simulink model "gm_sampleModel1467_3_sub"  (R2023a)
settings: Solver=VariableStepAuto  StartTime=0.0  StopTime=10.0  RelTol=1e-3
libraries: simulink x1
settings Model: Creator=user1  LastModifiedBy=user1
settings OptimizationCC: BlockReduction=off  ConditionallyExecuteInputs=off
settings DebuggingCC: InheritedTsInSrcMsg=none

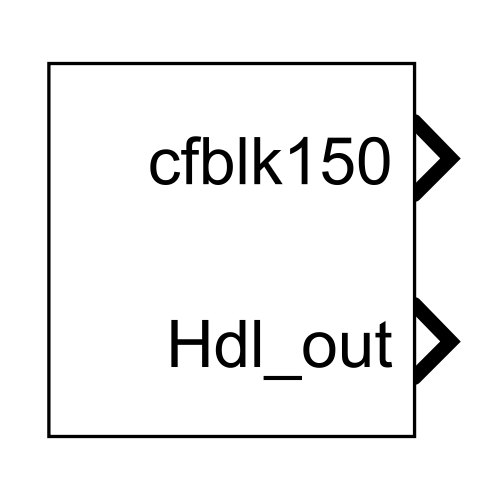
[thumbnail: Simulink's stored preview of the top-level diagram]
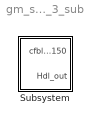
== system gm_sampleModel1467_3_sub ==
  Subsystem : Subsystem

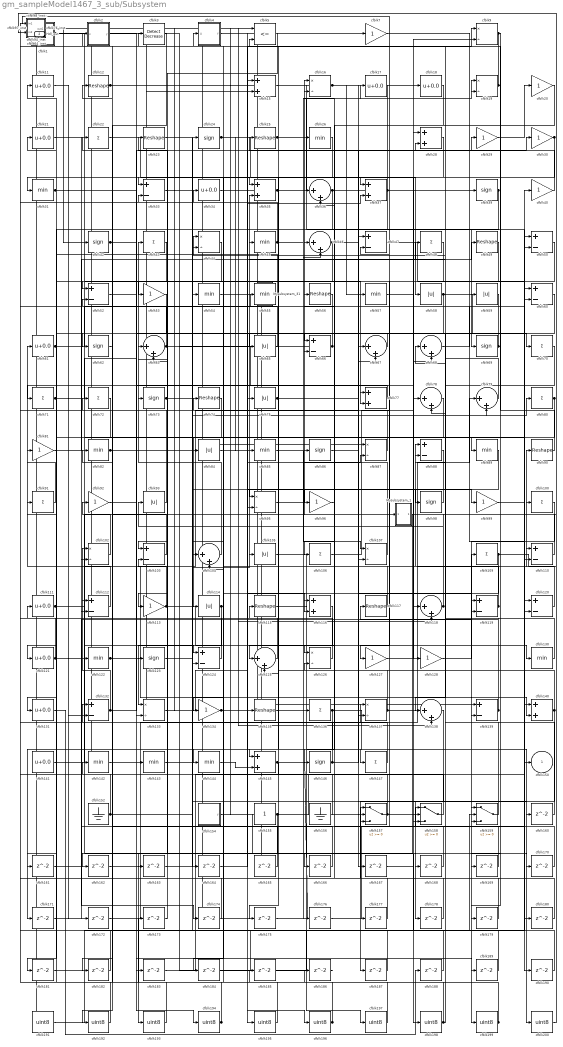
== system gm_sampleModel1467_3_sub/Subsystem ==
  Mysubsystem_1 : Subsystem
  Mysubsystem_31 : Subsystem
  cfblk1 : Subsystem  mask(Compare To Constant){relop=<=, const=double(3), OutDataTypeStr=uint8, ZeroCross=on}
      mask prompts: relop "Simulink:masks:Operator_MP"; const "Simulink:masks:ConstantValue_MP"; OutDataTypeStr "Simulink:masks:OutputDataType_MP"; ZeroCross "Simulink:masks:EnableZerocrossingDetection_MP"
      mask help: Simulink:masks:CompareToConstant_MD
      mask init:
      | OutDataTypeStr = 'uint8';
      | ZeroCross = 'on';
      | blkName = 'sampleModel1467_3_sub/Subsystem/cfblk1';
      | const = double(3);
      | const_str = '3.0';
      | const_val = double(3);
      | relop = '<=';
      | setValue = 'fixdt(0, 8)';
      | str = '<= 3';
      mask TypeOptions relop: == | ~= | < | <= | >= | >
      mask TypeOptions OutDataTypeStr: Simulink:masks:uint8 | Simulink:masks:boolean
      mask Callback ZeroCross: sl('zeroCrossEnable', gcbh);
      mask Display: disp(str)
  cfblk{22,43,48,70..72,80,91,100,106,109,136,147} (13 alike) : Sum  Inputs=+  OutDataTypeStr=uint8
  cfblk101_inst : Subsystem
  cfblk{9,16,19,44,87,95,102,107,126,133,137} (11 alike) : Product  Inputs=*/  OutDataTypeStr=uint8  RndMeth=Zero  SaturateOnIntegerOverflow=on
  cfblk{33,47,50,52,60,66,88,103,110,112,119..120,124,132,139} (15 alike) : Sum  Inputs=+-  OutDataTypeStr=uint8
  cfblk{36,46,63,67..68,78..79,104,118,125,138} (11 alike) : Sum  Inputs=|++  OutDataTypeStr=uint8
  cfblk{58..59,65,75,84,93,105,114} (8 alike) : Abs  OutDataTypeStr=uint8  SaturateOnIntegerOverflow=off
  cfblk{11,17..18,21,34,61,111,121,131,141} (10 alike) : Bias  Bias=0.0  SaturateOnIntegerOverflow=off
  cfblk{7,20,29..30,40,53,81,92,96,99,113,127..128,134} (14 alike) : Gain  OutDataTypeStr=uint8
  cfblk{12,23,25,49,56,74,90,115,117,135} (10 alike) : Reshape
  cfblk{15,28,35,37,77,116,140,145} (8 alike) : Sum  OutDataTypeStr=uint8
  cfblk{26,31,45,54..55,57,82,85,89,122,130,142..144} (14 alike) : MinMax  OutDataTypeStr=uint8
  cfblk{24,39,42,62,69,73,86,98,123,146} (10 alike) : Signum
  cfblk13_inst : Subsystem
  cfblk14_inst : Subsystem
  cfblk152 : Ground
  cfblk154 : Subsystem  mask(Counter Free-Running){NumBits=double(16), tsamp=double(-1)}
      mask prompts: NumBits "Simulink:masks:NumberOfBits_MP"; tsamp "Simulink:masks:SampleTime_MP"
      mask help: Simulink:masks:CounterFreeRunning_MD
  cfblk155 : Constant  OutDataTypeStr=uint8  SampleTime=-1
  cfblk156 : Ground
  cfblk157 : Switch  OutDataTypeStr=uint8  SaturateOnIntegerOverflow=off  InputSameDT=off
  cfblk158 : Switch  OutDataTypeStr=uint8  SaturateOnIntegerOverflow=off  InputSameDT=off
  cfblk159 : Switch  OutDataTypeStr=uint8  SaturateOnIntegerOverflow=off  InputSameDT=off
  cfblk{160..190} (31 alike) : Delay  SampleTime=1
  cfblk{191..200} (10 alike) : DataTypeConversion  OutDataTypeStr=uint8  SaturateOnIntegerOverflow=off  RndMeth=Floor
  cfblk2 : Subsystem  mask(Compare To Constant){relop=<=, const=double(3), OutDataTypeStr=uint8, ZeroCross=on}
      mask prompts: relop "Simulink:masks:Operator_MP"; const "Simulink:masks:ConstantValue_MP"; OutDataTypeStr "Simulink:masks:OutputDataType_MP"; ZeroCross "Simulink:masks:EnableZerocrossingDetection_MP"
      mask help: Simulink:masks:CompareToConstant_MD
      mask init:
      | OutDataTypeStr = 'uint8';
      | ZeroCross = 'on';
      | blkName = 'sampleModel1467_3_sub/Subsystem/cfblk2';
      | const = double(3);
      | const_str = '3.0';
      | const_val = double(3);
      | relop = '<=';
      | setValue = 'fixdt(0, 8)';
      | str = '<= 3';
      mask TypeOptions relop: == | ~= | < | <= | >= | >
      mask TypeOptions OutDataTypeStr: Simulink:masks:uint8 | Simulink:masks:boolean
      mask Callback ZeroCross: sl('zeroCrossEnable', gcbh);
      mask Display: disp(str)
  cfblk3 : simulink/Logic and Bit Operations/Detect Decrease  vinit=0.0  OutDataTypeStr=uint8
      settings: LibrarySourceBlock=|
      | hdlsllib/Logic and Bit
      | Operations/Detect
      | Decrease
  cfblk32_inst : Subsystem
  cfblk38_inst : Subsystem
  cfblk4 : Subsystem  mask(Detect Fall Nonpositive){vinit=double(0), InputProcessing=Elements as channels (sample based), OutDataTypeStr=uint8}
      mask prompts: vinit "Simulink:masks:InitialCondition_MP"; InputProcessing "Simulink:masks:InputProcessing_MP"; OutDataTypeStr "Simulink:masks:OutputDataType_MP"
      mask help: Simulink:masks:DetectFallNonpositive_MD
      mask init:
      | InputProcessing = 'Elements as channels (sample based)';
      | OutDataTypeStr = 'uint8';
      | vinit = double(0);
      mask TypeOptions InputProcessing: Simulink:masks:ColumnsAsChannelsFrameBased | Simulink:masks:ElementsAsChannelsSampleBased
      mask TypeOptions OutDataTypeStr: Simulink:masks:uint8 | Simulink:masks:boolean
      mask Display: fprintf('U <= 0\n&  NOT\nU/z <= 0')
  cfblk41_inst : Subsystem
  cfblk5 : RelationalOperator  Operator=<=  OutDataTypeStr=boolean  InputSameDT=off
  cfblk51_inst : Subsystem
  cfblk64_inst : Subsystem
  cfblk6_inst : Subsystem
  cfblk76_inst : Subsystem
  cfblk8_inst : Subsystem
  cfblk94_inst : Subsystem
  cfblk97_inst : Subsystem
  cfblk150 : Outport  OutDataTypeStr=uint8  SampleTime=1  VectorParamsAs1DForOutWhenUnconnected=off
  Hdl_out : Outport  Port=2  OutDataTypeStr=uint8  SampleTime=1
  wires:
  Mysubsystem_1/1(Out1) -> cfblk162/1
  Mysubsystem_31/1(Out1) -> cfblk165/1
  cfblk1/1(y) -> cfblk77/2, cfblk124/1
  cfblk100/1 -> cfblk199/1
  cfblk101_inst/1(out1) -> cfblk15/2, cfblk135/1
  cfblk102/1 -> cfblk92/1
  cfblk103/1 -> cfblk12/1
  cfblk104/1 -> cfblk43/1
  cfblk105/1 -> cfblk197/1
  cfblk106/1 -> cfblk14_inst/1(in1)
  cfblk107/1 -> cfblk16/1
  cfblk109/1 -> cfblk14_inst/2(in2), cfblk144/1
  cfblk11/1 -> cfblk172/1
  cfblk110/1 -> cfblk74/1
  cfblk111/1 -> cfblk66/2, cfblk200/1
  cfblk112/1 -> cfblk61/1
  cfblk113/1 -> cfblk103/2, cfblk130/1
  cfblk114/1 -> cfblk34/1, cfblk133/1
  cfblk115/1 -> cfblk147/1
  cfblk116/1 -> cfblk125/1
  cfblk117/1 -> cfblk35/2
  cfblk118/1 -> cfblk93/1, cfblk6_inst/2(in2)
  cfblk119/1 -> cfblk88/1, cfblk56/1, cfblk13_inst/1(in1)
  cfblk12/1 -> cfblk116/2, cfblk89/1
  cfblk120/1 -> cfblk90/1
  cfblk121/1 -> cfblk8_inst/1(in1), cfblk67/2
  cfblk122/1 -> cfblk47/1, cfblk139/2
  cfblk123/1 -> cfblk105/1
  cfblk124/1 -> cfblk38_inst/1(in1)
  cfblk125/1 -> cfblk22/1
  cfblk126/1 -> cfblk82/1
  cfblk127/1 -> cfblk68/2
  cfblk128/1 -> cfblk109/1
  cfblk13_inst/1(out1) -> cfblk7/1, cfblk136/1
  cfblk130/1 -> cfblk3/1
  cfblk131/1 -> cfblk188/1
  cfblk132/1 -> cfblk102/1, Mysubsystem_31/1(In1)
  cfblk133/1 -> cfblk55/1
  cfblk134/1 -> cfblk37/2, cfblk30/1
  cfblk135/1 -> cfblk17/1
  cfblk136/1 -> cfblk171/1, cfblk170/1
  cfblk137/1 -> cfblk79/1, cfblk46/1
  cfblk138/1 -> cfblk187/1
  cfblk139/1 -> cfblk117/1, cfblk44/1
  cfblk14_inst/1(out1) -> cfblk138/2
  cfblk140/1 -> cfblk73/1, cfblk178/1
  cfblk141/1 -> cfblk24/1
  cfblk142/1 -> cfblk86/1
  cfblk143/1 -> cfblk160/1
  cfblk144/1 -> cfblk145/2
  cfblk145/1 -> cfblk176/1, cfblk175/1
  cfblk146/1 -> cfblk5/2, cfblk29/1
  cfblk147/1 -> cfblk64_inst/2(in2)
  cfblk15/1 -> cfblk180/1
  cfblk152/1 -> cfblk8_inst/2(in2), cfblk124/2
  cfblk154/1(y) -> cfblk198/1
  cfblk155/1 -> cfblk193/1, cfblk40/1
  cfblk156/1 -> cfblk51_inst/1(in1)
  cfblk157/1 -> cfblk15/1, cfblk115/1
  cfblk158/1 -> cfblk142/1
  cfblk159/1 -> cfblk94_inst/1(in1)
  cfblk16/1 -> cfblk159/3, cfblk57/1
  cfblk160/1 -> cfblk126/2
  cfblk161/1 -> cfblk158/1
  cfblk162/1 -> cfblk107/2
  cfblk163/1 -> cfblk60/2
  cfblk164/1 -> cfblk87/2
  cfblk165/1 -> cfblk132/1
  cfblk166/1 -> cfblk63/1
  cfblk167/1 -> cfblk78/1
  cfblk168/1 -> cfblk36/2
  cfblk169/1 -> cfblk157/1
  cfblk17/1 -> cfblk33/1
  cfblk170/1 -> cfblk47/2
  cfblk171/1 -> cfblk119/2
  cfblk172/1 -> cfblk110/1
  cfblk173/1 -> cfblk33/2
  cfblk174/1 -> cfblk52/2
  cfblk175/1 -> cfblk137/1
  cfblk176/1 -> cfblk120/2
  cfblk177/1 -> cfblk94_inst/2(in2)
  cfblk178/1 -> cfblk157/3
  cfblk179/1 -> cfblk16/2
  cfblk18/1 -> cfblk146/1
  cfblk180/1 -> cfblk64_inst/1(in1)
  cfblk181/1 -> cfblk50/1
  cfblk182/1 -> cfblk41_inst/2(in2)
  cfblk183/1 -> cfblk46/2
  cfblk184/1 -> cfblk159/2
  cfblk185/1 -> cfblk158/3
  cfblk186/1 -> cfblk1/1(u)
  cfblk187/1 -> cfblk112/1
  cfblk188/1 -> cfblk32_inst/1(in1)
  cfblk189/1 -> cfblk38_inst/2(in2)
  cfblk19/1 -> cfblk13_inst/2(in2), cfblk169/1
  cfblk190/1 -> cfblk68/1
  cfblk191/1 -> cfblk54/1
  cfblk192/1 -> cfblk97_inst/1(in1)
  cfblk193/1 -> cfblk97_inst/2(in2)
  cfblk194/1 -> cfblk11/1, cfblk173/1
  cfblk195/1 -> cfblk2/1(u)
  cfblk196/1 -> cfblk111/1, cfblk186/1
  cfblk197/1 -> cfblk4/1(U)
  cfblk198/1 -> cfblk88/2, cfblk76_inst/2(in2)
  cfblk199/1 -> cfblk185/1, cfblk91/1
  cfblk2/1(y) -> cfblk194/1
  cfblk20/1 -> cfblk137/2
  cfblk200/1 -> cfblk100/1
  cfblk21/1 -> cfblk174/1
  cfblk22/1 -> cfblk75/1
  cfblk23/1 -> cfblk140/2
  cfblk24/1 -> cfblk58/1, cfblk128/1, cfblk85/1
  cfblk25/1 -> cfblk67/1, cfblk28/2
  cfblk26/1 -> cfblk145/1
  cfblk28/1 -> cfblk37/1
  cfblk29/1 -> cfblk20/1
  cfblk3/1 -> cfblk192/1
  cfblk30/1 -> cfblk104/2, cfblk163/1
  cfblk31/1 -> cfblk183/1, cfblk122/1
  cfblk32_inst/1(out1) -> cfblk18/1, cfblk118/2
  cfblk33/1 -> cfblk35/1
  cfblk34/1 -> cfblk195/1
  cfblk35/1 -> cfblk69/1, cfblk19/1
  cfblk36/1 -> cfblk63/2, cfblk44/2, cfblk133/2, Mysubsystem_1/1(In1)
  cfblk37/1 -> cfblk184/1, cfblk31/1
  cfblk38_inst/1(out1) -> cfblk141/1
  cfblk39/1 -> cfblk121/1, cfblk116/1
  cfblk4/1(Y) -> cfblk196/1
  cfblk40/1 -> cfblk25/1
  cfblk41_inst/1(out1) -> cfblk5/1, cfblk36/1
  cfblk42/1 -> cfblk189/1, cfblk70/1
  cfblk43/1 -> cfblk52/1
  cfblk44/1 -> cfblk181/1
  cfblk45/1 -> cfblk51_inst/2(in2), cfblk19/2
  cfblk46/1 -> cfblk119/1, cfblk102/2
  cfblk47/1 -> cfblk120/1
  cfblk48/1 -> cfblk134/1
  cfblk49/1 -> cfblk96/1
  cfblk5/1 -> cfblk53/1
  cfblk50/1 -> cfblk127/1
  cfblk51_inst/1(out1) -> cfblk177/1
  cfblk52/1 -> cfblk77/1
  cfblk53/1 -> cfblk161/1
  cfblk54/1 -> cfblk9/1
  cfblk55/1 -> cfblk21/1
  cfblk56/1 -> cfblk123/1
  cfblk57/1 -> cfblk9/2
  cfblk58/1 -> cfblk140/1, cfblk125/2, cfblk113/1
  cfblk59/1 -> cfblk78/2
  cfblk6_inst/1(out1) -> cfblk39/1
  cfblk60/1 -> cfblk126/1
  cfblk61/1 -> cfblk50/2, cfblk150/1
  cfblk62/1 -> cfblk182/1
  cfblk63/1 -> cfblk32_inst/2(in2), cfblk118/1
  cfblk64_inst/1(out1) -> cfblk42/1, cfblk87/1
  cfblk65/1 -> cfblk23/1
  cfblk66/1 -> cfblk65/1, Hdl_out/1
  cfblk67/1 -> cfblk62/1
  cfblk68/1 -> cfblk60/1
  cfblk69/1 -> cfblk66/1, cfblk179/1
  cfblk7/1 -> cfblk110/2
  cfblk70/1 -> cfblk138/1
  cfblk71/1 -> cfblk28/1, cfblk132/2, cfblk164/1
  cfblk72/1 -> cfblk131/1
  cfblk73/1 -> cfblk98/1, cfblk79/2, cfblk103/1
  cfblk74/1 -> cfblk114/1
  cfblk75/1 -> cfblk168/1, cfblk167/1
  cfblk76_inst/1(out1) -> cfblk6_inst/1(in1)
  cfblk77/1 -> cfblk71/1
  cfblk78/1 -> cfblk84/1
  cfblk79/1 -> cfblk45/1
  cfblk8_inst/1(out1) -> cfblk139/1, cfblk101_inst/1(in1)
  cfblk80/1 -> cfblk112/2, cfblk104/1
  cfblk81/1 -> cfblk48/1
  cfblk82/1 -> cfblk159/1, cfblk99/1
  cfblk84/1 -> cfblk80/1
  cfblk85/1 -> cfblk107/1
  cfblk86/1 -> cfblk157/2
  cfblk87/1 -> cfblk41_inst/1(in1)
  cfblk88/1 -> cfblk106/1
  cfblk89/1 -> cfblk95/1
  cfblk9/1 -> cfblk59/1, cfblk101_inst/2(in2)
  cfblk90/1 -> cfblk76_inst/1(in1)
  cfblk91/1 -> cfblk81/1
  cfblk92/1 -> cfblk166/1
  cfblk93/1 -> cfblk72/1
  cfblk94_inst/1(out1) -> cfblk158/2, cfblk143/1
  cfblk95/1 -> cfblk49/1
  cfblk96/1 -> cfblk26/1
  cfblk97_inst/1(out1) -> cfblk191/1
  cfblk98/1 -> cfblk95/2
  cfblk99/1 -> cfblk190/1

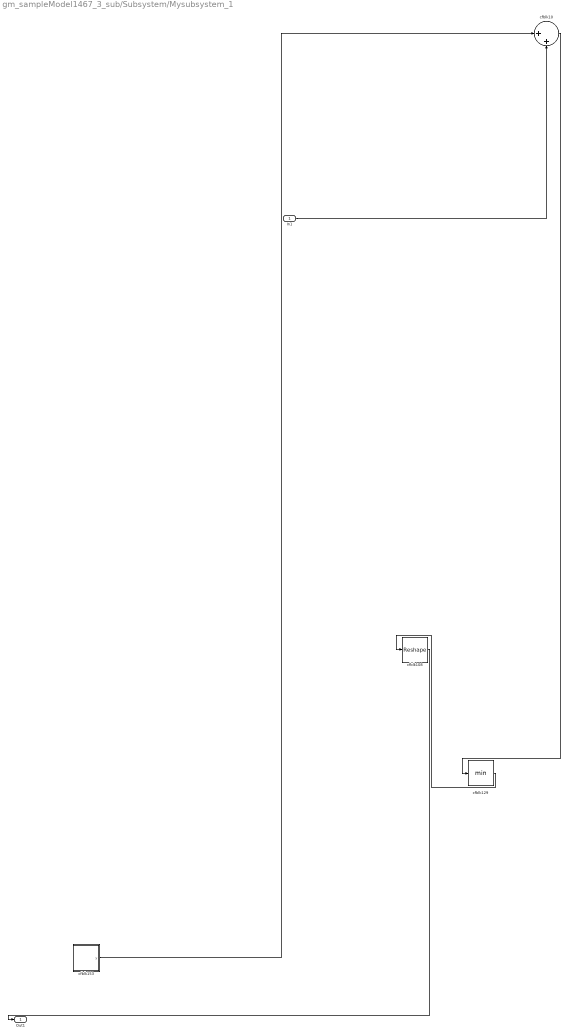
== system gm_sampleModel1467_3_sub/Subsystem/Mysubsystem_1 ==
  In1 : Inport  OutDataTypeStr=uint8  PortDimensions=1  SampleTime=1
  cfblk10 : Sum  Inputs=|++
  cfblk108 : Reshape
  cfblk129 : MinMax
  cfblk153 : Subsystem  mask(Counter Free-Running){NumBits=double(16), tsamp=double(-1)}
      mask prompts: NumBits "Simulink:masks:NumberOfBits_MP"; tsamp "Simulink:masks:SampleTime_MP"
      mask help: Simulink:masks:CounterFreeRunning_MD
  Out1 : Outport  SampleTime=1
  wires:
  In1/1 -> cfblk10/2
  cfblk10/1 -> cfblk129/1
  cfblk108/1 -> Out1/1
  cfblk129/1 -> cfblk108/1
  cfblk153/1(y) -> cfblk10/1

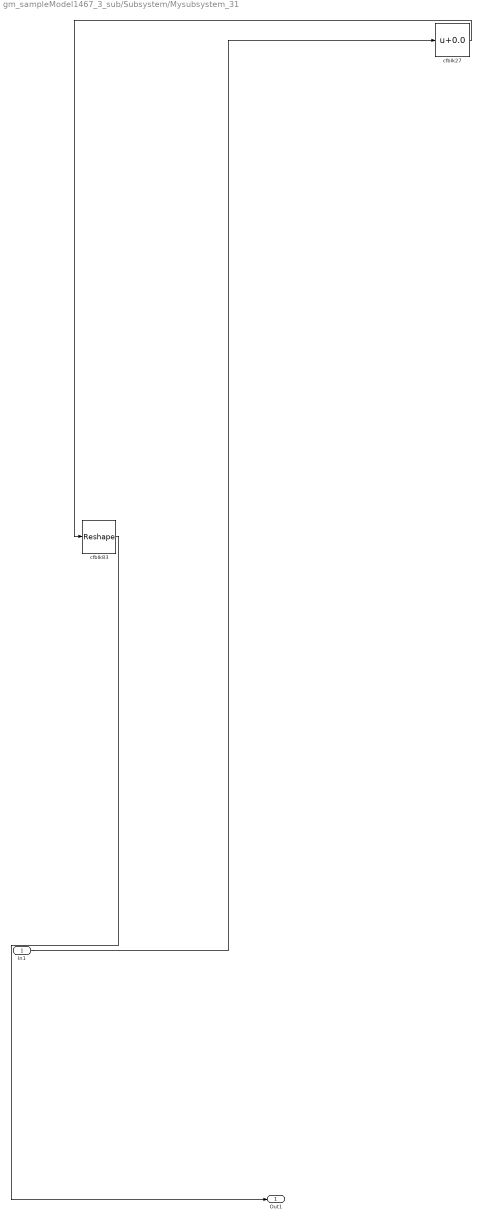
== system gm_sampleModel1467_3_sub/Subsystem/Mysubsystem_31 ==
  In1 : Inport  OutDataTypeStr=uint8  PortDimensions=1  SampleTime=1
  cfblk27 : Bias  Bias=0.0  SaturateOnIntegerOverflow=off
  cfblk83 : Reshape
  Out1 : Outport  SampleTime=1
  wires:
  In1/1 -> cfblk27/1
  cfblk27/1 -> cfblk83/1
  cfblk83/1 -> Out1/1

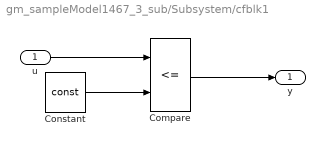
== system gm_sampleModel1467_3_sub/Subsystem/cfblk1 ==
  u : Inport  OutDataTypeStr=uint8  SampleTime=1
  Compare : RelationalOperator  Operator=<=  OutDataTypeStr=fixdt(0, 8)
  Constant : Constant  DisableCoverage=on  Value=const  OutDataTypeStr=Inherit: Inherit via back propagation  SampleTime=-1
  y : Outport  SampleTime=1
  wires:
  u/1 -> Compare/1
  Compare/1 -> y/1
  Constant/1 -> Compare/2

== system gm_sampleModel1467_3_sub/Subsystem/cfblk101_inst ==
  in1 : Inport  OutDataTypeStr=uint8  SampleTime=1
  in2 : Inport  Port=2  OutDataTypeStr=uint8  SampleTime=1
  mul_cfblk101_dotp_mulcomp : Product  Inputs=**  OutDataTypeStr=uint8  SampleTime=1
  out1 : Outport  OutDataTypeStr=uint8  SampleTime=1
  wires:
  in1/1 -> mul_cfblk101_dotp_mulcomp/1
  in2/1 -> mul_cfblk101_dotp_mulcomp/2
  mul_cfblk101_dotp_mulcomp/1 -> out1/1

== system gm_sampleModel1467_3_sub/Subsystem/cfblk13_inst ==
  in1 : Inport  OutDataTypeStr=uint8  SampleTime=1
  in2 : Inport  Port=2  OutDataTypeStr=uint8  SampleTime=1
  mul_cfblk13_dotp_mulcomp : Product  Inputs=**  OutDataTypeStr=uint8  SampleTime=1
  out1 : Outport  OutDataTypeStr=uint8  SampleTime=1
  wires:
  in1/1 -> mul_cfblk13_dotp_mulcomp/1
  in2/1 -> mul_cfblk13_dotp_mulcomp/2
  mul_cfblk13_dotp_mulcomp/1 -> out1/1

== system gm_sampleModel1467_3_sub/Subsystem/cfblk14_inst ==
  in1 : Inport  OutDataTypeStr=uint8  SampleTime=1
  in2 : Inport  Port=2  OutDataTypeStr=uint8  SampleTime=1
  mul_cfblk14_dotp_mulcomp : Product  Inputs=**  OutDataTypeStr=uint8  SampleTime=1
  out1 : Outport  OutDataTypeStr=uint8  SampleTime=1
  wires:
  in1/1 -> mul_cfblk14_dotp_mulcomp/1
  in2/1 -> mul_cfblk14_dotp_mulcomp/2
  mul_cfblk14_dotp_mulcomp/1 -> out1/1

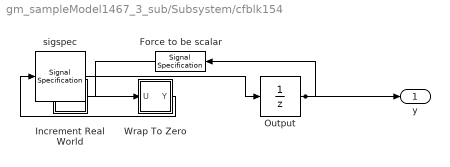
== system gm_sampleModel1467_3_sub/Subsystem/cfblk154 ==
  Force to be scalar : SignalSpecification  DisableCoverage=on  Dimensions=1
  Increment Real World : Subsystem  mask(Real World Value Increment){}
      mask help: Simulink:masks:RealWorldValueIncrement_MD
      mask Display: disp('V++')
  Output : UnitDelay  InitialCondition=0.0  SampleTime=tsamp  HasFrameUpgradeWarning=on
  Wrap To Zero : Subsystem  mask(Wrap To Zero){Threshold=double(65535)}
      mask prompts: Threshold "Simulink:masks:Threshold_MP"
      mask help: Simulink:masks:WrapToZero_MD
  sigspec : SignalSpecification  OutDataTypeStr=uint16  Dimensions=1
  y : Outport  SampleTime=1
  wires:
  Force to be scalar/1 -> Increment Real World/1(u)
  Increment Real World/1(y) -> Wrap To Zero/1(U)
  Output/1 -> Force to be scalar/1, y/1
  Wrap To Zero/1(Y) -> sigspec/1
  sigspec/1 -> Output/1

== system gm_sampleModel1467_3_sub/Subsystem/cfblk2 ==
  u : Inport  OutDataTypeStr=uint8  SampleTime=1
  Compare : RelationalOperator  Operator=<=  OutDataTypeStr=fixdt(0, 8)
  Constant : Constant  DisableCoverage=on  Value=const  OutDataTypeStr=Inherit: Inherit via back propagation  SampleTime=-1
  y : Outport  SampleTime=1
  wires:
  u/1 -> Compare/1
  Compare/1 -> y/1
  Constant/1 -> Compare/2

== system gm_sampleModel1467_3_sub/Subsystem/cfblk32_inst ==
  in1 : Inport  OutDataTypeStr=uint8  SampleTime=1
  in2 : Inport  Port=2  OutDataTypeStr=uint8  SampleTime=1
  mul_cfblk32_dotp_mulcomp : Product  Inputs=**  OutDataTypeStr=uint8  SampleTime=1
  out1 : Outport  OutDataTypeStr=uint8  SampleTime=1
  wires:
  in1/1 -> mul_cfblk32_dotp_mulcomp/1
  in2/1 -> mul_cfblk32_dotp_mulcomp/2
  mul_cfblk32_dotp_mulcomp/1 -> out1/1

== system gm_sampleModel1467_3_sub/Subsystem/cfblk38_inst ==
  in1 : Inport  OutDataTypeStr=uint8  SampleTime=1
  in2 : Inport  Port=2  OutDataTypeStr=uint8  SampleTime=1
  mul_cfblk38_dotp_mulcomp : Product  Inputs=**  OutDataTypeStr=uint8  SampleTime=1
  out1 : Outport  OutDataTypeStr=uint8  SampleTime=1
  wires:
  in1/1 -> mul_cfblk38_dotp_mulcomp/1
  in2/1 -> mul_cfblk38_dotp_mulcomp/2
  mul_cfblk38_dotp_mulcomp/1 -> out1/1

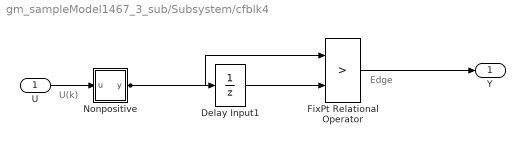
== system gm_sampleModel1467_3_sub/Subsystem/cfblk4 ==
  note: U(k)
  note: Edge
  U : Inport  OutDataTypeStr=uint8  SampleTime=1
  Delay Input1 : UnitDelay  Description=Store in Global RAM  DisableCoverage=on  InitialCondition=vinit  SampleTime=-1  HasFrameUpgradeWarning=on
  FixPt Relational Operator : RelationalOperator  Operator=>  OutDataTypeStr=fixdt(0, 8)  ZeroCross=off  InputSameDT=off
  Nonpositive : Subsystem  mask(Compare To Zero){relop=<=, OutDataTypeStr=boolean, ZeroCross=off}
      mask prompts: relop "Simulink:masks:Operator_MP"; OutDataTypeStr "Simulink:masks:OutputDataType_MP"; ZeroCross "Simulink:masks:EnableZerocrossingDetection_MP"
      mask help: Simulink:masks:CompareToZero_MD
      mask init:
      | OutDataTypeStr = 'boolean';
      | ZeroCross = 'off';
      | blkName = 'sampleModel1467_3_sub/Subsystem/cfblk4/Nonpositive';
      | relop = '<=';
      | setValue = 'boolean';
      mask TypeOptions relop: == | ~= | < | <= | >= | >
      mask TypeOptions OutDataTypeStr: Simulink:masks:uint8 | Simulink:masks:boolean
      mask Callback ZeroCross: sl('zeroCrossEnable', gcbh);
      mask Display: disp([relop,' 0'])
  Y : Outport  SampleTime=1
  wires:
  U/1 -> Nonpositive/1(u)
  Delay Input1/1 -> FixPt Relational Operator/2
  FixPt Relational Operator/1 -> Y/1
  Nonpositive/1(y) -> FixPt Relational Operator/1, Delay Input1/1

== system gm_sampleModel1467_3_sub/Subsystem/cfblk41_inst ==
  in1 : Inport  OutDataTypeStr=uint8  SampleTime=1
  in2 : Inport  Port=2  OutDataTypeStr=uint8  SampleTime=1
  mul_cfblk41_dotp_mulcomp : Product  Inputs=**  OutDataTypeStr=uint8  SampleTime=1
  out1 : Outport  OutDataTypeStr=uint8  SampleTime=1
  wires:
  in1/1 -> mul_cfblk41_dotp_mulcomp/1
  in2/1 -> mul_cfblk41_dotp_mulcomp/2
  mul_cfblk41_dotp_mulcomp/1 -> out1/1

== system gm_sampleModel1467_3_sub/Subsystem/cfblk51_inst ==
  in1 : Inport  OutDataTypeStr=uint8  SampleTime=1
  in2 : Inport  Port=2  OutDataTypeStr=uint8  SampleTime=1
  mul_cfblk51_dotp_mulcomp : Product  Inputs=**  OutDataTypeStr=uint8  SampleTime=1
  out1 : Outport  OutDataTypeStr=uint8  SampleTime=1
  wires:
  in1/1 -> mul_cfblk51_dotp_mulcomp/1
  in2/1 -> mul_cfblk51_dotp_mulcomp/2
  mul_cfblk51_dotp_mulcomp/1 -> out1/1

== system gm_sampleModel1467_3_sub/Subsystem/cfblk64_inst ==
  in1 : Inport  OutDataTypeStr=uint8  SampleTime=1
  in2 : Inport  Port=2  OutDataTypeStr=uint8  SampleTime=1
  mul_cfblk64_dotp_mulcomp : Product  Inputs=**  OutDataTypeStr=uint8  SampleTime=1
  out1 : Outport  OutDataTypeStr=uint8  SampleTime=1
  wires:
  in1/1 -> mul_cfblk64_dotp_mulcomp/1
  in2/1 -> mul_cfblk64_dotp_mulcomp/2
  mul_cfblk64_dotp_mulcomp/1 -> out1/1

== system gm_sampleModel1467_3_sub/Subsystem/cfblk6_inst ==
  in1 : Inport  OutDataTypeStr=uint8  SampleTime=1
  in2 : Inport  Port=2  OutDataTypeStr=uint8  SampleTime=1
  mul_cfblk6_dotp_mulcomp : Product  Inputs=**  OutDataTypeStr=uint8  SampleTime=1
  out1 : Outport  OutDataTypeStr=uint8  SampleTime=1
  wires:
  in1/1 -> mul_cfblk6_dotp_mulcomp/1
  in2/1 -> mul_cfblk6_dotp_mulcomp/2
  mul_cfblk6_dotp_mulcomp/1 -> out1/1

== system gm_sampleModel1467_3_sub/Subsystem/cfblk76_inst ==
  in1 : Inport  OutDataTypeStr=uint8  SampleTime=1
  in2 : Inport  Port=2  OutDataTypeStr=uint8  SampleTime=1
  mul_cfblk76_dotp_mulcomp : Product  Inputs=**  OutDataTypeStr=uint8  SampleTime=1
  out1 : Outport  OutDataTypeStr=uint8  SampleTime=1
  wires:
  in1/1 -> mul_cfblk76_dotp_mulcomp/1
  in2/1 -> mul_cfblk76_dotp_mulcomp/2
  mul_cfblk76_dotp_mulcomp/1 -> out1/1

== system gm_sampleModel1467_3_sub/Subsystem/cfblk8_inst ==
  in1 : Inport  OutDataTypeStr=uint8  SampleTime=1
  in2 : Inport  Port=2  OutDataTypeStr=uint8  SampleTime=1
  mul_cfblk8_dotp_mulcomp : Product  Inputs=**  OutDataTypeStr=uint8  SampleTime=1
  out1 : Outport  OutDataTypeStr=uint8  SampleTime=1
  wires:
  in1/1 -> mul_cfblk8_dotp_mulcomp/1
  in2/1 -> mul_cfblk8_dotp_mulcomp/2
  mul_cfblk8_dotp_mulcomp/1 -> out1/1

== system gm_sampleModel1467_3_sub/Subsystem/cfblk94_inst ==
  in1 : Inport  OutDataTypeStr=uint8  SampleTime=1
  in2 : Inport  Port=2  OutDataTypeStr=uint8  SampleTime=1
  mul_cfblk94_dotp_mulcomp : Product  Inputs=**  OutDataTypeStr=uint8  SampleTime=1
  out1 : Outport  OutDataTypeStr=uint8  SampleTime=1
  wires:
  in1/1 -> mul_cfblk94_dotp_mulcomp/1
  in2/1 -> mul_cfblk94_dotp_mulcomp/2
  mul_cfblk94_dotp_mulcomp/1 -> out1/1

== system gm_sampleModel1467_3_sub/Subsystem/cfblk97_inst ==
  in1 : Inport  OutDataTypeStr=uint8  SampleTime=1
  in2 : Inport  Port=2  OutDataTypeStr=uint8  SampleTime=1
  mul_cfblk97_dotp_mulcomp : Product  Inputs=**  OutDataTypeStr=uint8  SampleTime=1
  out1 : Outport  OutDataTypeStr=uint8  SampleTime=1
  wires:
  in1/1 -> mul_cfblk97_dotp_mulcomp/1
  in2/1 -> mul_cfblk97_dotp_mulcomp/2
  mul_cfblk97_dotp_mulcomp/1 -> out1/1

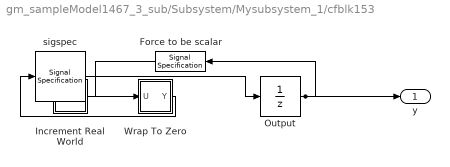
== system gm_sampleModel1467_3_sub/Subsystem/Mysubsystem_1/cfblk153 ==
  Force to be scalar : SignalSpecification  DisableCoverage=on  Dimensions=1
  Increment Real World : Subsystem  mask(Real World Value Increment){}
      mask help: Simulink:masks:RealWorldValueIncrement_MD
      mask Display: disp('V++')
  Output : UnitDelay  InitialCondition=0.0  SampleTime=tsamp  HasFrameUpgradeWarning=on
  Wrap To Zero : Subsystem  mask(Wrap To Zero){Threshold=double(65535)}
      mask prompts: Threshold "Simulink:masks:Threshold_MP"
      mask help: Simulink:masks:WrapToZero_MD
  sigspec : SignalSpecification  OutDataTypeStr=uint16  Dimensions=1
  y : Outport  SampleTime=1
  wires:
  Force to be scalar/1 -> Increment Real World/1(u)
  Increment Real World/1(y) -> Wrap To Zero/1(U)
  Output/1 -> Force to be scalar/1, y/1
  Wrap To Zero/1(Y) -> sigspec/1
  sigspec/1 -> Output/1

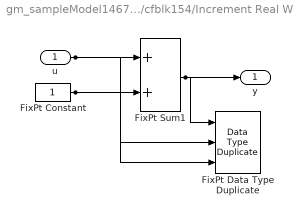
== system gm_sampleModel1467_3_sub/Subsystem/cfblk154/Increment Real World ==
  u : Inport  OutDataTypeStr=uint16  SampleTime=1
  FixPt Constant : Constant  DisableCoverage=on  OutDataTypeStr=Inherit: Inherit via back propagation  SampleTime=-1
  FixPt Data Type Duplicate : DataTypeDuplicate  DisableCoverage=on  NumInputPorts=3
  FixPt Sum1 : Sum  InputSameDT=on  OutDataTypeStr=Inherit: Inherit via back propagation  LockScale=on
  y : Outport  SampleTime=1
  wires:
  u/1 -> FixPt Sum1/1, FixPt Data Type Duplicate/2
  FixPt Constant/1 -> FixPt Sum1/2, FixPt Data Type Duplicate/3
  FixPt Sum1/1 -> FixPt Data Type Duplicate/1, y/1

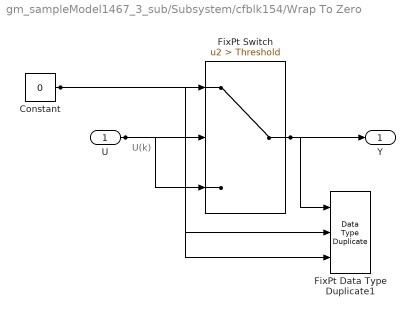
== system gm_sampleModel1467_3_sub/Subsystem/cfblk154/Wrap To Zero ==
  note: U(k)
  U : Inport  OutDataTypeStr=uint16  SampleTime=1
  Constant : Constant  DisableCoverage=on  Value=0  OutDataTypeStr=Inherit: Inherit via back propagation  SampleTime=-1
  FixPt Data Type Duplicate1 : DataTypeDuplicate  DisableCoverage=on  NumInputPorts=3
  FixPt Switch : Switch  Criteria=u2 > Threshold  Threshold=Threshold  OutDataTypeStr=Inherit: Inherit via back propagation  ZeroCross=off  SaturateOnIntegerOverflow=off  InputSameDT=off
  Y : Outport  SampleTime=1
  wires:
  U/1 -> FixPt Switch/3, FixPt Switch/2, FixPt Data Type Duplicate1/2
  Constant/1 -> FixPt Switch/1, FixPt Data Type Duplicate1/3
  FixPt Switch/1 -> FixPt Data Type Duplicate1/1, Y/1

== system gm_sampleModel1467_3_sub/Subsystem/cfblk4/Nonpositive ==
  u : Inport  OutDataTypeStr=uint8  SampleTime=1
  Compare : RelationalOperator  Operator=<=  OutDataTypeStr=boolean  ZeroCross=off
  Constant : Constant  DisableCoverage=on  Value=0  OutDataTypeStr=Inherit: Inherit via back propagation  SampleTime=-1  PreserveConstantTs=on
  y : Outport  SampleTime=1
  wires:
  u/1 -> Compare/1
  Compare/1 -> y/1
  Constant/1 -> Compare/2

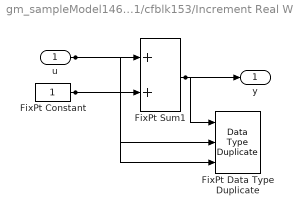
== system gm_sampleModel1467_3_sub/Subsystem/Mysubsystem_1/cfblk153/Increment Real World ==
  u : Inport  OutDataTypeStr=uint16  SampleTime=1
  FixPt Constant : Constant  DisableCoverage=on  OutDataTypeStr=Inherit: Inherit via back propagation  SampleTime=-1
  FixPt Data Type Duplicate : DataTypeDuplicate  DisableCoverage=on  NumInputPorts=3
  FixPt Sum1 : Sum  InputSameDT=on  OutDataTypeStr=Inherit: Inherit via back propagation  LockScale=on
  y : Outport  SampleTime=1
  wires:
  u/1 -> FixPt Sum1/1, FixPt Data Type Duplicate/2
  FixPt Constant/1 -> FixPt Sum1/2, FixPt Data Type Duplicate/3
  FixPt Sum1/1 -> FixPt Data Type Duplicate/1, y/1

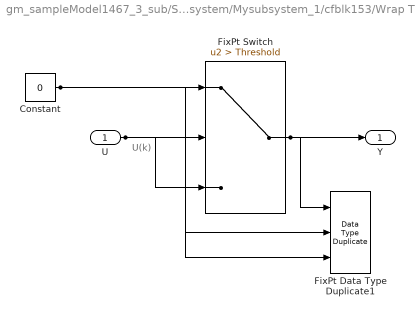
== system gm_sampleModel1467_3_sub/Subsystem/Mysubsystem_1/cfblk153/Wrap To Zero ==
  note: U(k)
  U : Inport  OutDataTypeStr=uint16  SampleTime=1
  Constant : Constant  DisableCoverage=on  Value=0  OutDataTypeStr=Inherit: Inherit via back propagation  SampleTime=-1
  FixPt Data Type Duplicate1 : DataTypeDuplicate  DisableCoverage=on  NumInputPorts=3
  FixPt Switch : Switch  Criteria=u2 > Threshold  Threshold=Threshold  OutDataTypeStr=Inherit: Inherit via back propagation  ZeroCross=off  SaturateOnIntegerOverflow=off  InputSameDT=off
  Y : Outport  SampleTime=1
  wires:
  U/1 -> FixPt Switch/3, FixPt Switch/2, FixPt Data Type Duplicate1/2
  Constant/1 -> FixPt Switch/1, FixPt Data Type Duplicate1/3
  FixPt Switch/1 -> FixPt Data Type Duplicate1/1, Y/1
